simulink model "CM340A_AdcDiagc"
settings: Solver=FixedStepDiscrete  SolverMode=SingleTasking  StartTime=0.0  StopTime=1  FixedStep=0.002  RelTol=1e-3
values from neighbouring files (symbols this model uses):
  Adc0Diagc = DataDict.NTC    [CM340A_AdcDiagc_DataDict.m]
  Adc1Diagc = DataDict.NTC    [CM340A_AdcDiagc_DataDict.m]
  ADCDIAG0REFVOLT_VOLT_F32 = DataDict.Constant    [CM340A_AdcDiagc_DataDict.m]
  ADCDIAG2REFVOLT_VOLT_F32 = DataDict.Constant    [CM340A_AdcDiagc_DataDict.m]
  ADCDIAG4REFVOLT_VOLT_F32 = DataDict.Constant    [CM340A_AdcDiagc_DataDict.m]
  AdcDiagcNtc0x032FailStep = DataDict.Calibration    [CM340A_AdcDiagc_DataDict.m]
  AdcDiagcNtc0x032PassStep = DataDict.Calibration    [CM340A_AdcDiagc_DataDict.m]
  AdcDiagcNtc0x033FailStep = DataDict.Calibration    [CM340A_AdcDiagc_DataDict.m]
  AdcDiagcNtc0x033PassStep = DataDict.Calibration    [CM340A_AdcDiagc_DataDict.m]
  AdcDiagcSt = DataDict.PIM    [CM340A_AdcDiagc_DataDict.m]
  ADCDIAGPARFLTPRM_CNT_U08 = DataDict.Constant    [CM340A_AdcDiagc_DataDict.m]
  ADCDIAGSCANGROUP2REFFLTPRM_CNT_U08 = DataDict.Constant    [CM340A_AdcDiagc_DataDict.m]
  ADCDIAGSCANGROUP3REFFLTPRM_CNT_U08 = DataDict.Constant    [CM340A_AdcDiagc_DataDict.m]
  ADCDIAGSCANGROUPENDREFVOLT_VOLT_F32 = DataDict.Constant    [CM340A_AdcDiagc_DataDict.m]
  ADCDIAGSCANGROUPSTRTREFVOLT_VOLT_F32 = DataDict.Constant    [CM340A_AdcDiagc_DataDict.m]
  ADCDNECRPARERRCLR_CNT_U08 = DataDict.Constant    [CM340A_AdcDiagc_DataDict.m]
  ADCDNPERPARERRMASK_CNT_U08 = DataDict.Constant    [CM340A_AdcDiagc_DataDict.m]
  VIRTCH21_CNT_U08 = DataDict.Constant    [CM340A_AdcDiagc_DataDict.m]
  VIRTCH22_CNT_U08 = DataDict.Constant    [CM340A_AdcDiagc_DataDict.m]
  VIRTCH23_CNT_U08 = DataDict.Constant    [CM340A_AdcDiagc_DataDict.m]
undefined symbols (not defined in the file or in its folder): NtcSts1, sigbuilder_block, SigQlfr1
libraries: simulink x42, CM340A_AdcDiagc_Library x40
(part 2 of 4)

== system CM340A_AdcDiagc/AdcDiagc/AdcDiagcPer1/NTC Fault Processing1 ==
  Adc1ParFlt : Inport
  Adc1 ParmByte : Inport  Port=2
  Add : Sum
  Atomic Subsystem : Subsystem  RequirementInfo="{'linktype_rmi_doors' '000079f2 (/ESG Group/FDD Module Requirements/EA4 Specific/CM340A_AdcDiagc)' '#CM340A_134' 'true' 'REQ:  CM340A_134' '' ; 'linktype_rmi_doors' '000079f2 (/ESG Group/FDD Module Requirements/EA4 Specific/CM340A_AdcDiagc)' '#CM340A_136' 'true' 'REQ:  CM340A_136' '' } %GIDa_bde32a42_2438_4464_b67f_8e12736c6683"  TreatAsAtomicUnit=on
  Constant3 : Constant  Value=Adc1Diagc
  CopyRight2 : Subsystem  Description=|  mask(Copyright Information){none=on}
      | Copyright info block.                                               
      |                                                                     
      | Place copyright information at the top of every subsystem in design.
      mask prompts: none "No parameters"
      mask help: Place copyright information at the top of every subsystem in design.
      mask Display:
      | NxtrConf = 'Nexteer Confidential';
      | 
      | sys = bdroot; %handle for the current model ("system")
      | first = get_param(sys,'Created');
      | first = first(end-3:end);  %year is last four digits
      | 
      | last = get_param(sys,'LastModifiedDate');
      | if isempty(last)
      |     last = datestr(now,'yyyy');
      | else
      |     last = last(end-3:end);
      | end
      | 
      | if strcmp(first,last)
      |     fprintf('%s -- Copyright %s Nexteer',NxtrConf,first)
      | else
      |     fprintf('%s -- %s%s- %s Nexteer',NxtrConf,char(169),first,last)
      | end
  Data Type Conversion : DataTypeConversion  OutDataTypeStr=Enum: SigQlfr1
  Data Type Conversion1 : DataTypeConversion  OutDataTypeStr=uint8
  Enumerated Constant : simulink/Sources/Enumerated Constant  OutDataTypeStr=Enum: SigQlfr1  Value=SigQlfr1.SIGQLFR_FAILD  SampleTime=inf
  GetNtcQlfr : Subsystem  RequirementInfo={} %GIDa_4498a704_80e4_4371_b34d_a62039516cac
  Relational Operator : RelationalOperator  Operator===  OutDataTypeStr=boolean
  SetNtcSts : Subsystem  RequirementInfo="{'linktype_rmi_doors' '000079f2 (/ESG Group/FDD Module Requirements/EA4 Specific/CM340A_AdcDiagc)' '#CM340A_130' 'true' 'REQ:  CM340A_130' '' } %GIDa_b72dd821_a9e1_4e8a_8139_63a1f2cdcabd"
  Adc1Faild : Outport
  wires:
  Relational Operator/1 -> Adc1Faild/1
  Enumerated Constant/1 -> Relational Operator/2
  Data Type Conversion/1 -> Relational Operator/1
  GetNtcQlfr/1(NtcQlfr) -> Data Type Conversion1/1
  Adc1 ParmByte/1 -> Add/1
  Atomic Subsystem/2(DebStep) -> SetNtcSts/4(DebStep)
  Atomic Subsystem/1(NtcSts) -> SetNtcSts/3(NtcSts)
  Constant3/1 -> GetNtcQlfr/1(NtcNr), SetNtcSts/1(NtcNr)  "NtcNr"
  Data Type Conversion1/1 -> Data Type Conversion/1
  Adc1ParFlt/1 -> Add/2
  Add/1 -> SetNtcSts/2(NtcStInfo), Atomic Subsystem/1(NtcStInfo)

== system CM340A_AdcDiagc/AdcDiagc/AdcDiagcPer1/Adc Daigc Pointer/CopyRight2 ==

== system CM340A_AdcDiagc/AdcDiagc/AdcDiagcPer1/Adc Daigc Pointer/Strt & End Ptr Output ==
  CopyRight2 : Subsystem  Description=|  mask(Copyright Information){none=on}
      | Copyright info block.                                               
      |                                                                     
      | Place copyright information at the top of every subsystem in design.
      mask prompts: none "No parameters"
      mask help: Place copyright information at the top of every subsystem in design.
      mask Display:
      | NxtrConf = 'Nexteer Confidential';
      | 
      | sys = bdroot; %handle for the current model ("system")
      | first = get_param(sys,'Created');
      | first = first(end-3:end);  %year is last four digits
      | 
      | last = get_param(sys,'LastModifiedDate');
      | if isempty(last)
      |     last = datestr(now,'yyyy');
      | else
      |     last = last(end-3:end);
      | end
      | 
      | if strcmp(first,last)
      |     fprintf('%s -- Copyright %s Nexteer',NxtrConf,first)
      | else
      |     fprintf('%s -- %s%s- %s Nexteer',NxtrConf,char(169),first,last)
      | end
  Data Store Read : DataStoreRead  DataStoreName=AdcDiagcStrtPtr
  Data Store Read1 : DataStoreRead  DataStoreName=AdcDiagcEndPtr
  AdcDiagcStrtPtr : Outport
  AdcDiagcEndPtr : Outport  Port=2
  wires:
  Data Store Read/1 -> AdcDiagcStrtPtr/1
  Data Store Read1/1 -> AdcDiagcEndPtr/1

== system CM340A_AdcDiagc/AdcDiagc/AdcDiagcPer1/Adc Daigc Pointer/Strt & End Ptr Store ==
  Adc Diag State : Inport
  CopyRight2 : Subsystem  Description=|  mask(Copyright Information){none=on}
      | Copyright info block.                                               
      |                                                                     
      | Place copyright information at the top of every subsystem in design.
      mask prompts: none "No parameters"
      mask help: Place copyright information at the top of every subsystem in design.
      mask Display:
      | NxtrConf = 'Nexteer Confidential';
      | 
      | sys = bdroot; %handle for the current model ("system")
      | first = get_param(sys,'Created');
      | first = first(end-3:end);  %year is last four digits
      | 
      | last = get_param(sys,'LastModifiedDate');
      | if isempty(last)
      |     last = datestr(now,'yyyy');
      | else
      |     last = last(end-3:end);
      | end
      | 
      | if strcmp(first,last)
      |     fprintf('%s -- Copyright %s Nexteer',NxtrConf,first)
      | else
      |     fprintf('%s -- %s%s- %s Nexteer',NxtrConf,char(169),first,last)
      | end
  Data Store Write : DataStoreWrite  DataStoreName=AdcDiagcStrtPtr
  Data Store Write1 : DataStoreWrite  DataStoreName=AdcDiagcEndPtr
  Merge : Merge  Inputs=4
  Merge1 : Merge  Inputs=4
  State 0 : Subsystem  RequirementInfo="{'linktype_rmi_doors' '000079f2 (/ESG Group/FDD Module Requirements/EA4 Specific/CM340A_AdcDiagc)' '#CM340A_189' 'true' 'REQ:  CM340A_189' '' } %GIDa_d7231089_39f2_44f7_8ddf_68c1ec68f84f"  TreatAsAtomicUnit=on
  State 1 : Subsystem  RequirementInfo="{'linktype_rmi_doors' '000079f2 (/ESG Group/FDD Module Requirements/EA4 Specific/CM340A_AdcDiagc)' '#CM340A_115' 'true' 'REQ:  CM340A_115' '' } %GIDa_53ce9ffd_18d8_43bb_bb31_5668534b0a0e"  TreatAsAtomicUnit=on
  State 2 : Subsystem  RequirementInfo="{'linktype_rmi_doors' '000079f2 (/ESG Group/FDD Module Requirements/EA4 Specific/CM340A_AdcDiagc)' '#CM340A_96' 'true' 'REQ:  CM340A_96' '' } %GIDa_d0356ceb_c141_4346_a11e_a54c0b3cccc5"  TreatAsAtomicUnit=on
  State 4 : Subsystem  RequirementInfo="{'linktype_rmi_doors' '000079f2 (/ESG Group/FDD Module Requirements/EA4 Specific/CM340A_AdcDiagc)' '#CM340A_106' 'true' 'REQ:  CM340A_106' '' } %GIDa_e4830bd7_ebc0_413b_b5ae_d9af4b1dd5b0"  TreatAsAtomicUnit=on
  State 6 : Subsystem  RequirementInfo="{'linktype_rmi_doors' '000079f2 (/ESG Group/FDD Module Requirements/EA4 Specific/CM340A_AdcDiagc)' '#CM340A_115' 'true' 'REQ:  CM340A_115' '' } %GIDa_697a9f40_2b37_43b7_b3e2_4ac1a7799fac"  TreatAsAtomicUnit=on
  State Based Determination1 : If  IfExpression=u1 == 0  ElseIfExpressions=u1 == 2, u1 == 4, u1 == 6
  wires:
  State Based Determination1/4 -> State 6/Action
  State 4/1(AdcDiagcStrtPtr) -> Merge/3
  State Based Determination1/1 -> State 0/Action
  State 0/1(AdcDiagcStrtPtr) -> Merge/1
  State Based Determination1/2 -> State 2/Action
  State 6/1(AdcDiagcStrtPtr) -> Merge/4
  Adc Diag State/1 -> State Based Determination1/1
  State 6/2(AdcDiagcEndPtr) -> Merge1/4
  Merge1/1 -> Data Store Write1/1
  State 2/1(AdcDiagcStrtPtr) -> Merge/2
  State 0/2(AdcDiagcEndPtr) -> Merge1/1
  State Based Determination1/3 -> State 4/Action
  Merge/1 -> Data Store Write/1
  State 2/2(AdcDiagcEndPtr) -> Merge1/2
  State 4/2(AdcDiagcEndPtr) -> Merge1/3
  State Based Determination1/5 -> State 1/Action

== system CM340A_AdcDiagc/AdcDiagc/AdcDiagcPer1/Adc Diag State/CopyRight2 ==

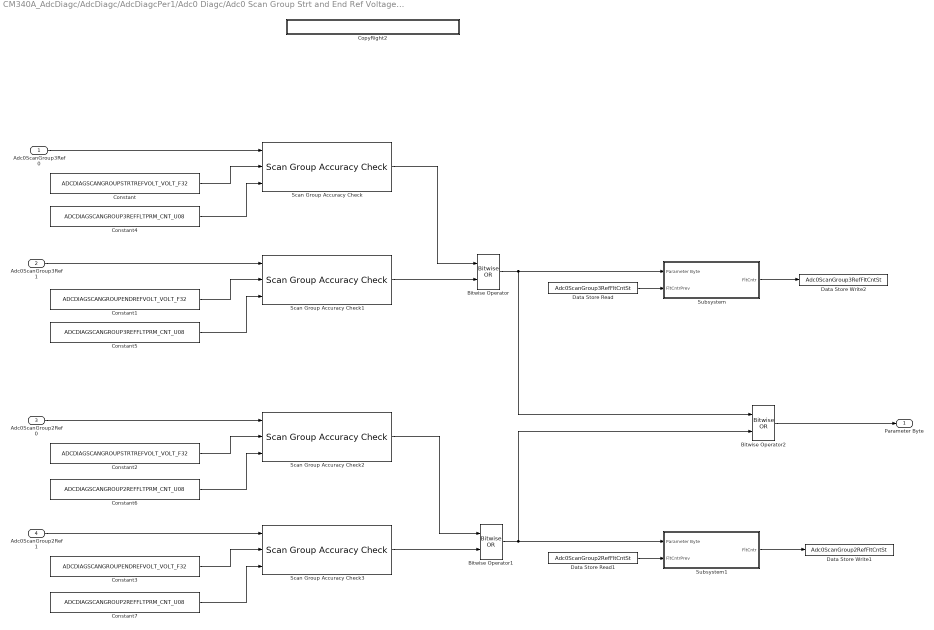
== system CM340A_AdcDiagc/AdcDiagc/AdcDiagcPer1/Adc0 Diagc/Adc0 Scan Group Strt and End Ref Voltage Diagc ==
  Adc0ScanGroup3Ref0 : Inport  RequirementInfo={} %GIDa_3923f31e_b6aa_43ec_bc9b_c94f6f317497
  Adc0ScanGroup3Ref1 : Inport  RequirementInfo={} %GIDa_ba8bf00c_f3fc_40d7_abef_0dabf128981a  Port=2
  Adc0ScanGroup2Ref0 : Inport  RequirementInfo={} %GIDa_6ca5502f_1ae3_4ae8_b00c_fe0941fa35eb  Port=3
  Adc0ScanGroup2Ref1 : Inport  RequirementInfo={} %GIDa_ae2e7cb2_cc28_4345_abb7_491be77205bd  Port=4
  Bitwise Operator : simulink/Logic and Bit Operations/Bitwise Operator  logicop=OR  UseBitMask=off  NumInputPorts=2  BitMask=bin2dec('11011001')  BitMaskRealWorld=Stored Integer
  Bitwise Operator1 : simulink/Logic and Bit Operations/Bitwise Operator  logicop=OR  UseBitMask=off  NumInputPorts=2  BitMask=bin2dec('11011001')  BitMaskRealWorld=Stored Integer
  Bitwise Operator2 : simulink/Logic and Bit Operations/Bitwise Operator  logicop=OR  UseBitMask=off  NumInputPorts=2  BitMask=bin2dec('11011001')  BitMaskRealWorld=Stored Integer
  Constant : Constant  Value=ADCDIAGSCANGROUPSTRTREFVOLT_VOLT_F32
  Constant1 : Constant  Value=ADCDIAGSCANGROUPENDREFVOLT_VOLT_F32
  Constant2 : Constant  Value=ADCDIAGSCANGROUPSTRTREFVOLT_VOLT_F32
  Constant3 : Constant  Value=ADCDIAGSCANGROUPENDREFVOLT_VOLT_F32
  Constant4 : Constant  Value=ADCDIAGSCANGROUP3REFFLTPRM_CNT_U08  OutDataTypeStr=uint8
  Constant5 : Constant  Value=ADCDIAGSCANGROUP3REFFLTPRM_CNT_U08  OutDataTypeStr=uint8
  Constant6 : Constant  Value=ADCDIAGSCANGROUP2REFFLTPRM_CNT_U08  OutDataTypeStr=uint8
  Constant7 : Constant  Value=ADCDIAGSCANGROUP2REFFLTPRM_CNT_U08  OutDataTypeStr=uint8
  CopyRight2 : Subsystem  Description=|  mask(Copyright Information){none=on}
      | Copyright info block.                                               
      |                                                                     
      | Place copyright information at the top of every subsystem in design.
      mask prompts: none "No parameters"
      mask help: Place copyright information at the top of every subsystem in design.
      mask Display:
      | NxtrConf = 'Nexteer Confidential';
      | 
      | sys = bdroot; %handle for the current model ("system")
      | first = get_param(sys,'Created');
      | first = first(end-3:end);  %year is last four digits
      | 
      | last = get_param(sys,'LastModifiedDate');
      | if isempty(last)
      |     last = datestr(now,'yyyy');
      | else
      |     last = last(end-3:end);
      | end
      | 
      | if strcmp(first,last)
      |     fprintf('%s -- Copyright %s Nexteer',NxtrConf,first)
      | else
      |     fprintf('%s -- %s%s- %s Nexteer',NxtrConf,char(169),first,last)
      | end
  Data Store Read : DataStoreRead  DataStoreName=Adc0ScanGroup3RefFltCntSt
  Data Store Read1 : DataStoreRead  DataStoreName=Adc0ScanGroup2RefFltCntSt
  Data Store Write1 : DataStoreWrite  DataStoreName=Adc0ScanGroup2RefFltCntSt
  Data Store Write2 : DataStoreWrite  DataStoreName=Adc0ScanGroup3RefFltCntSt
  Scan Group Accuracy Check{,1..3} (4 alike) : CM340A_AdcDiagc_Library/Scan Group Accuracy Check
  Subsystem : Subsystem
  Subsystem1 : Subsystem
  Parameter Byte : Outport
  wires:
  Adc0ScanGroup3Ref0/1 -> Scan Group Accuracy Check/1
  Constant/1 -> Scan Group Accuracy Check/2
  Adc0ScanGroup3Ref1/1 -> Scan Group Accuracy Check1/1
  Constant1/1 -> Scan Group Accuracy Check1/2
  Adc0ScanGroup2Ref0/1 -> Scan Group Accuracy Check2/1
  Constant2/1 -> Scan Group Accuracy Check2/2
  Scan Group Accuracy Check/1 -> Bitwise Operator/1
  Scan Group Accuracy Check1/1 -> Bitwise Operator/2
  Bitwise Operator/1 -> Bitwise Operator2/1, Subsystem/1(Parameter Byte)
  Adc0ScanGroup2Ref1/1 -> Scan Group Accuracy Check3/1
  Constant3/1 -> Scan Group Accuracy Check3/2
  Scan Group Accuracy Check3/1 -> Bitwise Operator1/2
  Bitwise Operator2/1 -> Parameter Byte/1
  Scan Group Accuracy Check2/1 -> Bitwise Operator1/1
  Constant4/1 -> Scan Group Accuracy Check/3
  Constant5/1 -> Scan Group Accuracy Check1/3
  Constant6/1 -> Scan Group Accuracy Check2/3
  Constant7/1 -> Scan Group Accuracy Check3/3
  Subsystem/1(FltCntr) -> Data Store Write2/1
  Bitwise Operator1/1 -> Subsystem1/1(Parameter Byte), Bitwise Operator2/2
  Data Store Read/1 -> Subsystem/2(FltCntrPrev)
  Data Store Read1/1 -> Subsystem1/2(FltCntrPrev)
  Subsystem1/1(FltCntr) -> Data Store Write1/1

== system CM340A_AdcDiagc/AdcDiagc/AdcDiagcPer1/Adc0 Diagc/CopyRight2 ==

== system CM340A_AdcDiagc/AdcDiagc/AdcDiagcPer1/Adc0 Diagc/State 0, 2, 4, 6 ==
  Adc0SelfDiag0 : Inport  RequirementInfo={} %GIDa_94e29999_33ff_4201_8add_daa4f5d70819
  Adc0SelfDiag2 : Inport  RequirementInfo={} %GIDa_c26eddb7_e945_49bf_b8c5_dde3d8ca2d62  Port=2
  Adc0SelfDiag4 : Inport  RequirementInfo={} %GIDa_06c9974f_8877_4a3b_918f_cfd71e4c9c58  Port=3
  Adc0DiagSt : Inport  RequirementInfo={} %GIDa_3045ed8c_f79b_488d_b603_a76a50a7acd0  Port=4
  Action Port : ActionPort  ActionType=case
  Merge : Merge  Inputs=4
  State 0 : Subsystem  RequirementInfo="{'linktype_rmi_doors' '000079f2 (/ESG Group/FDD Module Requirements/EA4 Specific/CM340A_AdcDiagc)' '#CM340A_189' 'true' 'REQ:  CM340A_189' '' } %GIDa_a6da38dc_83ca_4031_acbe_834917661ebd"  TreatAsAtomicUnit=on
  State 2 : Subsystem  RequirementInfo="{'linktype_rmi_doors' '000079f2 (/ESG Group/FDD Module Requirements/EA4 Specific/CM340A_AdcDiagc)' '#CM340A_96' 'true' 'REQ:  CM340A_96' '' } %GIDa_33825e2f_213e_4946_b631_0cc3f71b8274"  TreatAsAtomicUnit=on
  State 4 : Subsystem  RequirementInfo="{'linktype_rmi_doors' '000079f2 (/ESG Group/FDD Module Requirements/EA4 Specific/CM340A_AdcDiagc)' '#CM340A_106' 'true' 'REQ:  CM340A_106' '' } %GIDa_cf9e8958_cd24_4cdd_ad67_cff793a850a5"  TreatAsAtomicUnit=on
  State 6 : Subsystem  RequirementInfo="{'linktype_rmi_doors' '000079f2 (/ESG Group/FDD Module Requirements/EA4 Specific/CM340A_AdcDiagc)' '#CM340A_115' 'true' 'REQ:  CM340A_115' '' } %GIDa_c79baab0_0759_49b6_a0c6_0635325daffc"  TreatAsAtomicUnit=on
  State Based Determination : If  IfExpression=u1 == 0  ElseIfExpressions=u1 == 2, u1 == 4
  Parameter Byte : Outport
  wires:
  Adc0DiagSt/1 -> State 2/4(DiagState), State 6/4(DiagState), State 4/4(DiagState), State 0/4(DiagState), State Based Determination/1
  Adc0SelfDiag0/1 -> State 6/1(Adc0SelfDiag0), State 4/1(Adc0SelfDiag0), State 2/1(Adc0SelfDiag0), State 0/1(Adc0SelfDiag0)
  Adc0SelfDiag2/1 -> State 6/2(Adc0SelfDiag2), State 4/2(Adc0SelfDiag2), State 2/2(Adc0SelfDiag2), State 0/2(Adc0SelfDiag2)
  Adc0SelfDiag4/1 -> State 6/3(Adc0SelfDiag4), State 4/3(Adc0SelfDiag4), State 2/3(Adc0SelfDiag4), State 0/3(Adc0SelfDiag4)
  State 0/1(Parameter Byte) -> Merge/1
  State 2/1(Parameter Byte) -> Merge/2
  State 4/1(Parameter Byte) -> Merge/3
  State 6/1(Parameter Byte) -> Merge/4
  Merge/1 -> Parameter Byte/1
  State Based Determination/1 -> State 0/Action
  State Based Determination/2 -> State 2/Action
  State Based Determination/3 -> State 4/Action
  State Based Determination/4 -> State 6/Action

== system CM340A_AdcDiagc/AdcDiagc/AdcDiagcPer1/Adc0 Diagc/State 1,3,5,7 ==
  Action Port : ActionPort  ActionType=default
  Constant : Constant  Value=0  OutDataTypeStr=uint8
  CopyRight2 : Subsystem  Description=|  mask(Copyright Information){none=on}
      | Copyright info block.                                               
      |                                                                     
      | Place copyright information at the top of every subsystem in design.
      mask prompts: none "No parameters"
      mask help: Place copyright information at the top of every subsystem in design.
      mask Display:
      | NxtrConf = 'Nexteer Confidential';
      | 
      | sys = bdroot; %handle for the current model ("system")
      | first = get_param(sys,'Created');
      | first = first(end-3:end);  %year is last four digits
      | 
      | last = get_param(sys,'LastModifiedDate');
      | if isempty(last)
      |     last = datestr(now,'yyyy');
      | else
      |     last = last(end-3:end);
      | end
      | 
      | if strcmp(first,last)
      |     fprintf('%s -- Copyright %s Nexteer',NxtrConf,first)
      | else
      |     fprintf('%s -- %s%s- %s Nexteer',NxtrConf,char(169),first,last)
      | end
  Parameter Byte : Outport
  wires:
  Constant/1 -> Parameter Byte/1

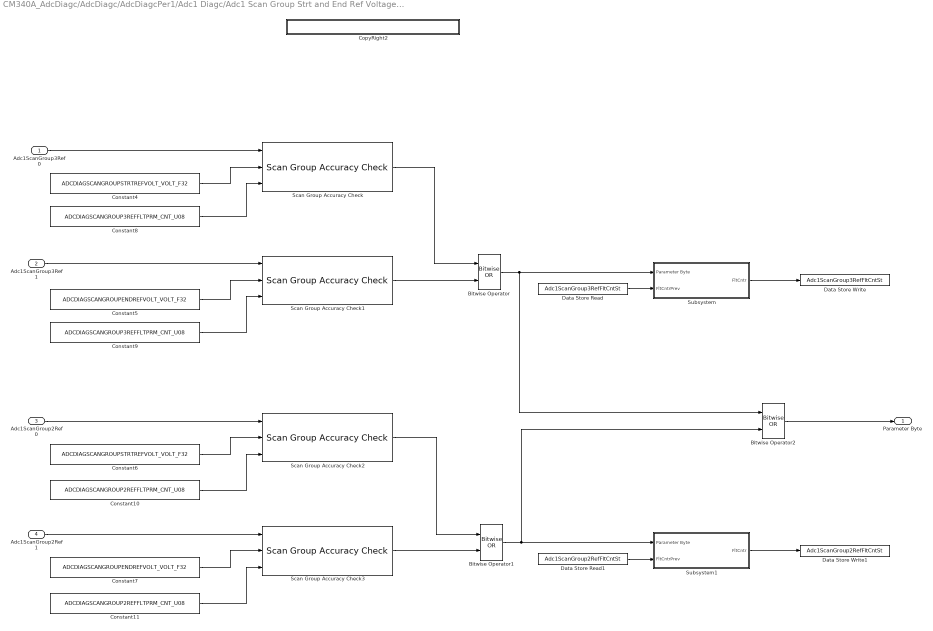
== system CM340A_AdcDiagc/AdcDiagc/AdcDiagcPer1/Adc1 Diagc/Adc1 Scan Group Strt and End Ref Voltage Diagc ==
  Adc1ScanGroup3Ref0 : Inport  RequirementInfo={} %GIDa_01845f96_04cc_48cb_8cdf_d81f529bf610
  Adc1ScanGroup3Ref1 : Inport  RequirementInfo={} %GIDa_d1be0a00_9783_4d18_831d_acb83b27fe4f  Port=2
  Adc1ScanGroup2Ref0 : Inport  RequirementInfo={} %GIDa_3fed8bb6_e00c_497f_b5bc_7887f6a81f53  Port=3
  Adc1ScanGroup2Ref1 : Inport  RequirementInfo={} %GIDa_4db4f757_00a1_4030_b70d_cb6c9e614cb5  Port=4
  Bitwise Operator : simulink/Logic and Bit Operations/Bitwise Operator  logicop=OR  UseBitMask=off  NumInputPorts=2  BitMask=bin2dec('11011001')  BitMaskRealWorld=Stored Integer
  Bitwise Operator1 : simulink/Logic and Bit Operations/Bitwise Operator  logicop=OR  UseBitMask=off  NumInputPorts=2  BitMask=bin2dec('11011001')  BitMaskRealWorld=Stored Integer
  Bitwise Operator2 : simulink/Logic and Bit Operations/Bitwise Operator  logicop=OR  UseBitMask=off  NumInputPorts=2  BitMask=bin2dec('11011001')  BitMaskRealWorld=Stored Integer
  Constant10 : Constant  Value=ADCDIAGSCANGROUP2REFFLTPRM_CNT_U08  OutDataTypeStr=uint8
  Constant11 : Constant  Value=ADCDIAGSCANGROUP2REFFLTPRM_CNT_U08  OutDataTypeStr=uint8
  Constant4 : Constant  Value=ADCDIAGSCANGROUPSTRTREFVOLT_VOLT_F32
  Constant5 : Constant  Value=ADCDIAGSCANGROUPENDREFVOLT_VOLT_F32
  Constant6 : Constant  Value=ADCDIAGSCANGROUPSTRTREFVOLT_VOLT_F32
  Constant7 : Constant  Value=ADCDIAGSCANGROUPENDREFVOLT_VOLT_F32
  Constant8 : Constant  Value=ADCDIAGSCANGROUP3REFFLTPRM_CNT_U08  OutDataTypeStr=uint8
  Constant9 : Constant  Value=ADCDIAGSCANGROUP3REFFLTPRM_CNT_U08  OutDataTypeStr=uint8
  CopyRight2 : Subsystem  Description=|  mask(Copyright Information){none=on}
      | Copyright info block.                                               
      |                                                                     
      | Place copyright information at the top of every subsystem in design.
      mask prompts: none "No parameters"
      mask help: Place copyright information at the top of every subsystem in design.
      mask Display:
      | NxtrConf = 'Nexteer Confidential';
      | 
      | sys = bdroot; %handle for the current model ("system")
      | first = get_param(sys,'Created');
      | first = first(end-3:end);  %year is last four digits
      | 
      | last = get_param(sys,'LastModifiedDate');
      | if isempty(last)
      |     last = datestr(now,'yyyy');
      | else
      |     last = last(end-3:end);
      | end
      | 
      | if strcmp(first,last)
      |     fprintf('%s -- Copyright %s Nexteer',NxtrConf,first)
      | else
      |     fprintf('%s -- %s%s- %s Nexteer',NxtrConf,char(169),first,last)
      | end
  Data Store Read : DataStoreRead  DataStoreName=Adc1ScanGroup3RefFltCntSt
  Data Store Read1 : DataStoreRead  DataStoreName=Adc1ScanGroup2RefFltCntSt
  Data Store Write : DataStoreWrite  DataStoreName=Adc1ScanGroup3RefFltCntSt
  Data Store Write1 : DataStoreWrite  DataStoreName=Adc1ScanGroup2RefFltCntSt
  Scan Group Accuracy Check{,1..3} (4 alike) : CM340A_AdcDiagc_Library/Scan Group Accuracy Check
  Subsystem : Subsystem
  Subsystem1 : Subsystem
  Parameter Byte : Outport
  wires:
  Scan Group Accuracy Check/1 -> Bitwise Operator/1
  Scan Group Accuracy Check1/1 -> Bitwise Operator/2
  Subsystem/1(FltCntr) -> Data Store Write/1
  Scan Group Accuracy Check2/1 -> Bitwise Operator1/1
  Scan Group Accuracy Check3/1 -> Bitwise Operator1/2
  Subsystem1/1(FltCntr) -> Data Store Write1/1
  Bitwise Operator2/1 -> Parameter Byte/1
  Adc1ScanGroup3Ref0/1 -> Scan Group Accuracy Check/1
  Constant4/1 -> Scan Group Accuracy Check/2
  Adc1ScanGroup3Ref1/1 -> Scan Group Accuracy Check1/1
  Constant5/1 -> Scan Group Accuracy Check1/2
  Adc1ScanGroup2Ref0/1 -> Scan Group Accuracy Check2/1
  Constant6/1 -> Scan Group Accuracy Check2/2
  Adc1ScanGroup2Ref1/1 -> Scan Group Accuracy Check3/1
  Constant7/1 -> Scan Group Accuracy Check3/2
  Constant8/1 -> Scan Group Accuracy Check/3
  Constant9/1 -> Scan Group Accuracy Check1/3
  Constant10/1 -> Scan Group Accuracy Check2/3
  Constant11/1 -> Scan Group Accuracy Check3/3
  Bitwise Operator/1 -> Subsystem/1(Parameter Byte), Bitwise Operator2/1
  Bitwise Operator1/1 -> Subsystem1/1(Parameter Byte), Bitwise Operator2/2
  Data Store Read/1 -> Subsystem/2(FltCntrPrev)
  Data Store Read1/1 -> Subsystem1/2(FltCntrPrev)

== system CM340A_AdcDiagc/AdcDiagc/AdcDiagcPer1/Adc1 Diagc/CopyRight2 ==

== system CM340A_AdcDiagc/AdcDiagc/AdcDiagcPer1/Adc1 Diagc/State 0,2,4,6 ==
  Adc1SelfDiag0 : Inport  RequirementInfo={} %GIDa_34a48fa0_dd63_46cc_bd9d_829bbe1f86cf
  Adc1SelfDiag2 : Inport  RequirementInfo={} %GIDa_4de6ae8c_be2f_440b_b497_7b7a185d7705  Port=2
  Adc1SelfDiag4 : Inport  RequirementInfo={} %GIDa_eacb0038_7c4f_43e2_bdc2_c657f83f78ba  Port=3
  Adc1DiagSt : Inport  RequirementInfo={} %GIDa_82c28b46_226d_4e6c_8857_1d9eb21c6cb5  Port=4
  Action Port : ActionPort  ActionType=case
  CopyRight2 : Subsystem  Description=|  mask(Copyright Information){none=on}
      | Copyright info block.                                               
      |                                                                     
      | Place copyright information at the top of every subsystem in design.
      mask prompts: none "No parameters"
      mask help: Place copyright information at the top of every subsystem in design.
      mask Display:
      | NxtrConf = 'Nexteer Confidential';
      | 
      | sys = bdroot; %handle for the current model ("system")
      | first = get_param(sys,'Created');
      | first = first(end-3:end);  %year is last four digits
      | 
      | last = get_param(sys,'LastModifiedDate');
      | if isempty(last)
      |     last = datestr(now,'yyyy');
      | else
      |     last = last(end-3:end);
      | end
      | 
      | if strcmp(first,last)
      |     fprintf('%s -- Copyright %s Nexteer',NxtrConf,first)
      | else
      |     fprintf('%s -- %s%s- %s Nexteer',NxtrConf,char(169),first,last)
      | end
  Merge : Merge  Inputs=4
  State 0 : Subsystem  RequirementInfo="{'linktype_rmi_doors' '000079f2 (/ESG Group/FDD Module Requirements/EA4 Specific/CM340A_AdcDiagc)' '#CM340A_200' 'true' 'REQ:  CM340A_200' '' } %GIDa_e35781c5_1e91_4292_ba5d_515a26f8b285"  TreatAsAtomicUnit=on
  State 2 : Subsystem  RequirementInfo="{'linktype_rmi_doors' '000079f2 (/ESG Group/FDD Module Requirements/EA4 Specific/CM340A_AdcDiagc)' '#CM340A_151' 'true' 'REQ:  CM340A_151' '' } %GIDa_47bc9f9e_be13_46f9_a398_ba75de96ec4b"  TreatAsAtomicUnit=on
  State 4 : Subsystem  RequirementInfo="{'linktype_rmi_doors' '000079f2 (/ESG Group/FDD Module Requirements/EA4 Specific/CM340A_AdcDiagc)' '#CM340A_160' 'true' 'REQ:  CM340A_160' '' } %GIDa_c894ce70_8a7d_498e_8eac_cd0715dd161e"  TreatAsAtomicUnit=on
  State 6 : Subsystem  RequirementInfo="{'linktype_rmi_doors' '000079f2 (/ESG Group/FDD Module Requirements/EA4 Specific/CM340A_AdcDiagc)' '#CM340A_169' 'true' 'REQ:  CM340A_169' '' } %GIDa_9580dbab_c802_4d44_ba6f_46aa79aa5561"  TreatAsAtomicUnit=on
  State Based Determination : If  IfExpression=u1 == 0  ElseIfExpressions=u1 == 2, u1 == 4
  Parameter Byte : Outport
  wires:
  Merge/1 -> Parameter Byte/1
  State 6/1(Parameter Byte) -> Merge/4
  State 4/1(Parameter Byte) -> Merge/3
  State 2/1(Parameter Byte) -> Merge/2
  State 0/1(Parameter Byte) -> Merge/1
  Adc1SelfDiag4/1 -> State 6/3(Adc1SelfDiag4), State 4/3(Adc1SelfDiag4), State 2/3(Adc1SelfDiag4), State 0/3(Adc1SelfDiag4)
  Adc1SelfDiag2/1 -> State 6/2(Adc1SelfDiag2), State 4/2(Adc1SelfDiag2), State 2/2(Adc1SelfDiag2), State 0/2(Adc1SelfDiag2)
  Adc1SelfDiag0/1 -> State 6/1(Adc1SelfDiag0), State 4/1(Adc1SelfDiag0), State 2/1(Adc1SelfDiag0), State 0/1(Adc1SelfDiag0)
  Adc1DiagSt/1 -> State 4/4(DiagState), State 6/4(DiagState), State 2/4(DiagState), State 0/4(DiagState), State Based Determination/1
  State Based Determination/1 -> State 0/Action
  State Based Determination/2 -> State 2/Action
  State Based Determination/3 -> State 4/Action
  State Based Determination/4 -> State 6/Action

== system CM340A_AdcDiagc/AdcDiagc/AdcDiagcPer1/Adc1 Diagc/State 1,3,5,7 ==
  Action Port : ActionPort  ActionType=default
  Constant : Constant  Value=0  OutDataTypeStr=uint8
  CopyRight2 : Subsystem  Description=|  mask(Copyright Information){none=on}
      | Copyright info block.                                               
      |                                                                     
      | Place copyright information at the top of every subsystem in design.
      mask prompts: none "No parameters"
      mask help: Place copyright information at the top of every subsystem in design.
      mask Display:
      | NxtrConf = 'Nexteer Confidential';
      | 
      | sys = bdroot; %handle for the current model ("system")
      | first = get_param(sys,'Created');
      | first = first(end-3:end);  %year is last four digits
      | 
      | last = get_param(sys,'LastModifiedDate');
      | if isempty(last)
      |     last = datestr(now,'yyyy');
      | else
      |     last = last(end-3:end);
      | end
      | 
      | if strcmp(first,last)
      |     fprintf('%s -- Copyright %s Nexteer',NxtrConf,first)
      | else
      |     fprintf('%s -- %s%s- %s Nexteer',NxtrConf,char(169),first,last)
      | end
  Parameter Byte : Outport
  wires:
  Constant/1 -> Parameter Byte/1

== system CM340A_AdcDiagc/AdcDiagc/AdcDiagcPer1/AdcDiagcPer2/CopyRight2 ==

== system CM340A_AdcDiagc/AdcDiagc/AdcDiagcPer1/AdcDiagcPer2/Set Adc0ParFlt 0 ==
  Action Port : ActionPort  ActionType=else
  CopyRight2 : Subsystem  Description=|  mask(Copyright Information){none=on}
      | Copyright info block.                                               
      |                                                                     
      | Place copyright information at the top of every subsystem in design.
      mask prompts: none "No parameters"
      mask help: Place copyright information at the top of every subsystem in design.
      mask Display:
      | NxtrConf = 'Nexteer Confidential';
      | 
      | sys = bdroot; %handle for the current model ("system")
      | first = get_param(sys,'Created');
      | first = first(end-3:end);  %year is last four digits
      | 
      | last = get_param(sys,'LastModifiedDate');
      | if isempty(last)
      |     last = datestr(now,'yyyy');
      | else
      |     last = last(end-3:end);
      | end
      | 
      | if strcmp(first,last)
      |     fprintf('%s -- Copyright %s Nexteer',NxtrConf,first)
      | else
      |     fprintf('%s -- %s%s- %s Nexteer',NxtrConf,char(169),first,last)
      | end
  zero : Constant  Value=0  OutDataTypeStr=uint8
  Adc1ParFlt : Outport
  wires:
  zero/1 -> Adc1ParFlt/1

== system CM340A_AdcDiagc/AdcDiagc/AdcDiagcPer1/AdcDiagcPer2/Set Adc0ParFlt to 0 ==
  Action Port : ActionPort  ActionType=else
  CopyRight2 : Subsystem  Description=|  mask(Copyright Information){none=on}
      | Copyright info block.                                               
      |                                                                     
      | Place copyright information at the top of every subsystem in design.
      mask prompts: none "No parameters"
      mask help: Place copyright information at the top of every subsystem in design.
      mask Display:
      | NxtrConf = 'Nexteer Confidential';
      | 
      | sys = bdroot; %handle for the current model ("system")
      | first = get_param(sys,'Created');
      | first = first(end-3:end);  %year is last four digits
      | 
      | last = get_param(sys,'LastModifiedDate');
      | if isempty(last)
      |     last = datestr(now,'yyyy');
      | else
      |     last = last(end-3:end);
      | end
      | 
      | if strcmp(first,last)
      |     fprintf('%s -- Copyright %s Nexteer',NxtrConf,first)
      | else
      |     fprintf('%s -- %s%s- %s Nexteer',NxtrConf,char(169),first,last)
      | end
  zero : Constant  Value=0  OutDataTypeStr=uint8
  Adc0ParFlt : Outport
  wires:
  zero/1 -> Adc0ParFlt/1

== system CM340A_AdcDiagc/AdcDiagc/AdcDiagcPer1/AdcDiagcPer2/Set Adc0ParFlt to 128 and Err Clr Reg to 2 ==
  note: This represents a Register Write not a software Output Variable
  Action Port : ActionPort  ActionType=then
  ADCDIAGPARFLTPRM_CNT_U08 : Constant  Value=ADCDIAGPARFLTPRM_CNT_U08  OutDataTypeStr=uint8
  ADCDIAGPARFLTPRM_CNT_U1 : Constant  Value=ADCDNECRPARERRCLR_CNT_U08  OutDataTypeStr=uint8
      settings: AttributesFormatString=%<OutDataTypeStr>
  CopyRight2 : Subsystem  Description=|  mask(Copyright Information){none=on}
      | Copyright info block.                                               
      |                                                                     
      | Place copyright information at the top of every subsystem in design.
      mask prompts: none "No parameters"
      mask help: Place copyright information at the top of every subsystem in design.
      mask Display:
      | NxtrConf = 'Nexteer Confidential';
      | 
      | sys = bdroot; %handle for the current model ("system")
      | first = get_param(sys,'Created');
      | first = first(end-3:end);  %year is last four digits
      | 
      | last = get_param(sys,'LastModifiedDate');
      | if isempty(last)
      |     last = datestr(now,'yyyy');
      | else
      |     last = last(end-3:end);
      | end
      | 
      | if strcmp(first,last)
      |     fprintf('%s -- Copyright %s Nexteer',NxtrConf,first)
      | else
      |     fprintf('%s -- %s%s- %s Nexteer',NxtrConf,char(169),first,last)
      | end
  RegOutpADCD0ECR : Terminator
  Adc0ParFlt : Outport
  wires:
  ADCDIAGPARFLTPRM_CNT_U08/1 -> Adc0ParFlt/1
  ADCDIAGPARFLTPRM_CNT_U1/1 -> RegOutpADCD0ECR/1

== system CM340A_AdcDiagc/AdcDiagc/AdcDiagcPer1/AdcDiagcPer2/Set Adc1ParFlt to 128 and Err Clr Reg to 4 ==
  note: This represents a Register Write not a software Output Variable
  Action Port : ActionPort  ActionType=then
  ADCDIAGPARFLTPRM_CNT_U08 : Constant  Value=ADCDIAGPARFLTPRM_CNT_U08  OutDataTypeStr=uint8
  ADCDIAGPARFLTPRM_CNT_U1 : Constant  Value=ADCDNECRPARERRCLR_CNT_U08  OutDataTypeStr=uint8
      settings: AttributesFormatString=%<OutDataTypeStr>
  CopyRight2 : Subsystem  Description=|  mask(Copyright Information){none=on}
      | Copyright info block.                                               
      |                                                                     
      | Place copyright information at the top of every subsystem in design.
      mask prompts: none "No parameters"
      mask help: Place copyright information at the top of every subsystem in design.
      mask Display:
      | NxtrConf = 'Nexteer Confidential';
      | 
      | sys = bdroot; %handle for the current model ("system")
      | first = get_param(sys,'Created');
      | first = first(end-3:end);  %year is last four digits
      | 
      | last = get_param(sys,'LastModifiedDate');
      | if isempty(last)
      |     last = datestr(now,'yyyy');
      | else
      |     last = last(end-3:end);
      | end
      | 
      | if strcmp(first,last)
      |     fprintf('%s -- Copyright %s Nexteer',NxtrConf,first)
      | else
      |     fprintf('%s -- %s%s- %s Nexteer',NxtrConf,char(169),first,last)
      | end
  RegOutpADCD1ECR : Terminator
  Adc1ParFlt : Outport
  wires:
  ADCDIAGPARFLTPRM_CNT_U08/1 -> Adc1ParFlt/1
  ADCDIAGPARFLTPRM_CNT_U1/1 -> RegOutpADCD1ECR/1

== system CM340A_AdcDiagc/AdcDiagc/AdcDiagcPer1/NTC Fault Processing0/Atomic Subsystem ==
  NtcStInfo : Inport  OutDataTypeStr=uint8
  CopyRight2 : Subsystem  Description=|  mask(Copyright Information){none=on}
      | Copyright info block.                                               
      |                                                                     
      | Place copyright information at the top of every subsystem in design.
      mask prompts: none "No parameters"
      mask help: Place copyright information at the top of every subsystem in design.
      mask Display:
      | NxtrConf = 'Nexteer Confidential';
      | 
      | sys = bdroot; %handle for the current model ("system")
      | first = get_param(sys,'Created');
      | first = first(end-3:end);  %year is last four digits
      | 
      | last = get_param(sys,'LastModifiedDate');
      | if isempty(last)
      |     last = datestr(now,'yyyy');
      | else
      |     last = last(end-3:end);
      | end
      | 
      | if strcmp(first,last)
      |     fprintf('%s -- Copyright %s Nexteer',NxtrConf,first)
      | else
      |     fprintf('%s -- %s%s- %s Nexteer',NxtrConf,char(169),first,last)
      | end
  Fail Step : Subsystem  TreatAsAtomicUnit=on
  If : If
  Merge : Merge
  Merge1 : Merge
  Pass Step : Subsystem  RequirementInfo={} %GIDa_f2406e4f_5e57_490d_8d1c_469ab90954f0  TreatAsAtomicUnit=on
  NtcSts : Outport
  DebStep : Outport  Port=2  OutDataTypeStr=uint16
  wires:
  NtcStInfo/1 -> If/1
  If/1 -> Fail Step/Action
  If/2 -> Pass Step/Action
  Merge/1 -> DebStep/1
  Fail Step/1(NtcSts) -> Merge1/1
  Pass Step/1(NtcSts) -> Merge1/2
  Merge1/1 -> NtcSts/1
  Fail Step/2(DebStep) -> Merge/1
  Pass Step/2(DebStep) -> Merge/2

== system CM340A_AdcDiagc/AdcDiagc/AdcDiagcPer1/NTC Fault Processing0/CopyRight2 ==

== system CM340A_AdcDiagc/AdcDiagc/AdcDiagcPer1/NTC Fault Processing0/GetNtcQlfr ==
  NtcNr : Inport
  CopyRight2 : Subsystem  Description=|  mask(Copyright Information){none=on}
      | Copyright info block.                                               
      |                                                                     
      | Place copyright information at the top of every subsystem in design.
      mask prompts: none "No parameters"
      mask help: Place copyright information at the top of every subsystem in design.
      mask Display:
      | NxtrConf = 'Nexteer Confidential';
      | 
      | sys = bdroot; %handle for the current model ("system")
      | first = get_param(sys,'Created');
      | first = first(end-3:end);  %year is last four digits
      | 
      | last = get_param(sys,'LastModifiedDate');
      | if isempty(last)
      |     last = datestr(now,'yyyy');
      | else
      |     last = last(end-3:end);
      | end
      | 
      | if strcmp(first,last)
      |     fprintf('%s -- Copyright %s Nexteer',NxtrConf,first)
      | else
      |     fprintf('%s -- %s%s- %s Nexteer',NxtrConf,char(169),first,last)
      | end
  Data Store Read : DataStoreRead  DataStoreName=Adc0DynDiagcQlfr
  Terminator : Terminator
  NtcQlfr : Outport
  wires:
  NtcNr/1 -> Terminator/1
  Data Store Read/1 -> NtcQlfr/1

== system CM340A_AdcDiagc/AdcDiagc/AdcDiagcPer1/NTC Fault Processing0/SetNtcSts ==
  note: Note:
      |
      | - "ISO Fault Debounce Design" Simulink block intent to use here for Simulation purpose only. Do not Code this block
  NtcNr : Inport
  NtcStInfo : Inport  Port=2
  NtcSts : Inport  Port=3  OutDataTypeStr=Enum: NtcSts1
  DebStep : Inport  Port=4
  CopyRight2 : Subsystem  Description=|  mask(Copyright Information){none=on}
      | Copyright info block.                                               
      |                                                                     
      | Place copyright information at the top of every subsystem in design.
      mask prompts: none "No parameters"
      mask help: Place copyright information at the top of every subsystem in design.
      mask Display:
      | NxtrConf = 'Nexteer Confidential';
      | 
      | sys = bdroot; %handle for the current model ("system")
      | first = get_param(sys,'Created');
      | first = first(end-3:end);  %year is last four digits
      | 
      | last = get_param(sys,'LastModifiedDate');
      | if isempty(last)
      |     last = datestr(now,'yyyy');
      | else
      |     last = last(end-3:end);
      | end
      | 
      | if strcmp(first,last)
      |     fprintf('%s -- Copyright %s Nexteer',NxtrConf,first)
      | else
      |     fprintf('%s -- %s%s- %s Nexteer',NxtrConf,char(169),first,last)
      | end
  Data Store Write : DataStoreWrite  DataStoreName=Adc0DynDiagcQlfr
  Data Type Conversion1 : DataTypeConversion  OutMin=0  OutMax=255  OutDataTypeStr=uint8
  Enabled Subsystem : Subsystem  TreatAsAtomicUnit=on
  Faild : Constant  Value=2
  Ground : Ground
  ISO Fault Debounce Design : Stateflow chart  TreatAsAtomicUnit=on
      settings: AttributesFormatString=|
      | Simulation Purpose Only.
      | Do Not Code this block
      | Diagnostic Manager Owns this requirement
  Relational Operator : RelationalOperator  Operator===  OutDataTypeStr=boolean
  Scope1 : Scope  NumInputPorts=5
      settings: YMin=-5~-5~-5~-5~-5  YMax=5~5~5~5~5  SaveName=ScopeData5
  Terminator : Terminator
  Terminator1 : Terminator
  wires:
  NtcStInfo/1 -> Scope1/4, Enabled Subsystem/1(In1), Terminator1/1
  NtcNr/1 -> Terminator/1
  NtcSts/1 -> Data Type Conversion1/1
  DebStep/1 -> ISO Fault Debounce Design/2(DebStep), Scope1/2
  ISO Fault Debounce Design/1(Qualifier) -> Relational Operator/1, Scope1/3, Data Store Write/1
  Ground/1 -> ISO Fault Debounce Design/3(SvcClr)
  Data Type Conversion1/1 -> ISO Fault Debounce Design/1(NtcSts), Scope1/1
  ISO Fault Debounce Design/2(ErrAccOut) -> Scope1/5
  Faild/1 -> Relational Operator/2
  Relational Operator/1 -> Enabled Subsystem/Enable

== system CM340A_AdcDiagc/AdcDiagc/AdcDiagcPer1/NTC Fault Processing1/Atomic Subsystem ==
  NtcStInfo : Inport  OutDataTypeStr=uint8
  CopyRight2 : Subsystem  Description=|  mask(Copyright Information){none=on}
      | Copyright info block.                                               
      |                                                                     
      | Place copyright information at the top of every subsystem in design.
      mask prompts: none "No parameters"
      mask help: Place copyright information at the top of every subsystem in design.
      mask Display:
      | NxtrConf = 'Nexteer Confidential';
      | 
      | sys = bdroot; %handle for the current model ("system")
      | first = get_param(sys,'Created');
      | first = first(end-3:end);  %year is last four digits
      | 
      | last = get_param(sys,'LastModifiedDate');
      | if isempty(last)
      |     last = datestr(now,'yyyy');
      | else
      |     last = last(end-3:end);
      | end
      | 
      | if strcmp(first,last)
      |     fprintf('%s -- Copyright %s Nexteer',NxtrConf,first)
      | else
      |     fprintf('%s -- %s%s- %s Nexteer',NxtrConf,char(169),first,last)
      | end
  Fail Step : Subsystem  TreatAsAtomicUnit=on
  If : If
  Merge : Merge
  Merge1 : Merge
  Pass Step : Subsystem  RequirementInfo={} %GIDa_8179ac39_d4c7_4151_9d94_184fec5ce1ce  TreatAsAtomicUnit=on
  NtcSts : Outport
  DebStep : Outport  Port=2  OutDataTypeStr=uint16
  wires:
  Pass Step/2(DebStep) -> Merge/2
  Fail Step/2(DebStep) -> Merge/1
  Merge1/1 -> NtcSts/1
  Pass Step/1(NtcSts) -> Merge1/2
  Fail Step/1(NtcSts) -> Merge1/1
  Merge/1 -> DebStep/1
  If/2 -> Pass Step/Action
  If/1 -> Fail Step/Action
  NtcStInfo/1 -> If/1

== system CM340A_AdcDiagc/AdcDiagc/AdcDiagcPer1/NTC Fault Processing1/CopyRight2 ==

== system CM340A_AdcDiagc/AdcDiagc/AdcDiagcPer1/NTC Fault Processing1/GetNtcQlfr ==
  NtcNr : Inport
  CopyRight2 : Subsystem  Description=|  mask(Copyright Information){none=on}
      | Copyright info block.                                               
      |                                                                     
      | Place copyright information at the top of every subsystem in design.
      mask prompts: none "No parameters"
      mask help: Place copyright information at the top of every subsystem in design.
      mask Display:
      | NxtrConf = 'Nexteer Confidential';
      | 
      | sys = bdroot; %handle for the current model ("system")
      | first = get_param(sys,'Created');
      | first = first(end-3:end);  %year is last four digits
      | 
      | last = get_param(sys,'LastModifiedDate');
      | if isempty(last)
      |     last = datestr(now,'yyyy');
      | else
      |     last = last(end-3:end);
      | end
      | 
      | if strcmp(first,last)
      |     fprintf('%s -- Copyright %s Nexteer',NxtrConf,first)
      | else
      |     fprintf('%s -- %s%s- %s Nexteer',NxtrConf,char(169),first,last)
      | end
  Data Store Read : DataStoreRead  DataStoreName=Adc1DynDiagcQlfr
  Terminator : Terminator
  NtcQlfr : Outport
  wires:
  Data Store Read/1 -> NtcQlfr/1
  NtcNr/1 -> Terminator/1

== system CM340A_AdcDiagc/AdcDiagc/AdcDiagcPer1/NTC Fault Processing1/SetNtcSts ==
  note: Note:
      |
      | - "ISO Fault Debounce Design" Simulink block intent to use here for Simulation purpose only. Do not Code this block
  NtcNr : Inport
  NtcStInfo : Inport  Port=2
  NtcSts : Inport  Port=3  OutDataTypeStr=Enum: NtcSts1
  DebStep : Inport  Port=4
  CopyRight2 : Subsystem  Description=|  mask(Copyright Information){none=on}
      | Copyright info block.                                               
      |                                                                     
      | Place copyright information at the top of every subsystem in design.
      mask prompts: none "No parameters"
      mask help: Place copyright information at the top of every subsystem in design.
      mask Display:
      | NxtrConf = 'Nexteer Confidential';
      | 
      | sys = bdroot; %handle for the current model ("system")
      | first = get_param(sys,'Created');
      | first = first(end-3:end);  %year is last four digits
      | 
      | last = get_param(sys,'LastModifiedDate');
      | if isempty(last)
      |     last = datestr(now,'yyyy');
      | else
      |     last = last(end-3:end);
      | end
      | 
      | if strcmp(first,last)
      |     fprintf('%s -- Copyright %s Nexteer',NxtrConf,first)
      | else
      |     fprintf('%s -- %s%s- %s Nexteer',NxtrConf,char(169),first,last)
      | end
  Data Store Write : DataStoreWrite  DataStoreName=Adc1DynDiagcQlfr
  Data Type Conversion1 : DataTypeConversion  OutMin=0  OutMax=255  OutDataTypeStr=uint8
  Enabled Subsystem : Subsystem  TreatAsAtomicUnit=on
  Faild : Constant  Value=2
  Ground : Ground
  ISO Fault Debounce Design : Stateflow chart  TreatAsAtomicUnit=on
      settings: AttributesFormatString=|
      | Simulation Purpose Only.
      | Do Not Code this block
      | Diagnostic Manager Owns this requirement
  Relational Operator : RelationalOperator  Operator===  OutDataTypeStr=boolean
  Scope1 : Scope  NumInputPorts=5
      settings: YMin=-5~-5~-5~-5~-5  YMax=5~5~5~5~5  SaveName=ScopeData5
  Terminator : Terminator
  Terminator1 : Terminator
  wires:
  ISO Fault Debounce Design/2(ErrAccOut) -> Scope1/5
  Data Type Conversion1/1 -> Scope1/1, ISO Fault Debounce Design/1(NtcSts)
  Ground/1 -> ISO Fault Debounce Design/3(SvcClr)
  DebStep/1 -> Scope1/2, ISO Fault Debounce Design/2(DebStep)
  NtcSts/1 -> Data Type Conversion1/1
  NtcNr/1 -> Terminator/1
  NtcStInfo/1 -> Terminator1/1, Enabled Subsystem/1(In1), Scope1/4
  ISO Fault Debounce Design/1(Qualifier) -> Data Store Write/1, Scope1/3, Relational Operator/1
  Faild/1 -> Relational Operator/2
  Relational Operator/1 -> Enabled Subsystem/Enable

== system CM340A_AdcDiagc/AdcDiagc/AdcDiagcPer1/Adc Daigc Pointer/Strt & End Ptr Output/CopyRight2 ==

== system CM340A_AdcDiagc/AdcDiagc/AdcDiagcPer1/Adc Daigc Pointer/Strt & End Ptr Store/CopyRight2 ==

== system CM340A_AdcDiagc/AdcDiagc/AdcDiagcPer1/Adc Daigc Pointer/Strt & End Ptr Store/State 0 ==
  Action Port : ActionPort  ActionType=then
  Constant3 : Constant  Value=VIRTCH22_CNT_U08
  Constant4 : Constant  Value=VIRTCH23_CNT_U08
  CopyRight2 : Subsystem  Description=|  mask(Copyright Information){none=on}
      | Copyright info block.                                               
      |                                                                     
      | Place copyright information at the top of every subsystem in design.
      mask prompts: none "No parameters"
      mask help: Place copyright information at the top of every subsystem in design.
      mask Display:
      | NxtrConf = 'Nexteer Confidential';
      | 
      | sys = bdroot; %handle for the current model ("system")
      | first = get_param(sys,'Created');
      | first = first(end-3:end);  %year is last four digits
      | 
      | last = get_param(sys,'LastModifiedDate');
      | if isempty(last)
      |     last = datestr(now,'yyyy');
      | else
      |     last = last(end-3:end);
      | end
      | 
      | if strcmp(first,last)
      |     fprintf('%s -- Copyright %s Nexteer',NxtrConf,first)
      | else
      |     fprintf('%s -- %s%s- %s Nexteer',NxtrConf,char(169),first,last)
      | end
  AdcDiagcStrtPtr : Outport
  AdcDiagcEndPtr : Outport  Port=2
  wires:
  Constant3/1 -> AdcDiagcStrtPtr/1
  Constant4/1 -> AdcDiagcEndPtr/1

== system CM340A_AdcDiagc/AdcDiagc/AdcDiagcPer1/Adc Daigc Pointer/Strt & End Ptr Store/State 1 ==
  note: /*Do Nothing*/
  Action Port : ActionPort  ActionType=else
  CopyRight2 : Subsystem  Description=|  mask(Copyright Information){none=on}
      | Copyright info block.                                               
      |                                                                     
      | Place copyright information at the top of every subsystem in design.
      mask prompts: none "No parameters"
      mask help: Place copyright information at the top of every subsystem in design.
      mask Display:
      | NxtrConf = 'Nexteer Confidential';
      | 
      | sys = bdroot; %handle for the current model ("system")
      | first = get_param(sys,'Created');
      | first = first(end-3:end);  %year is last four digits
      | 
      | last = get_param(sys,'LastModifiedDate');
      | if isempty(last)
      |     last = datestr(now,'yyyy');
      | else
      |     last = last(end-3:end);
      | end
      | 
      | if strcmp(first,last)
      |     fprintf('%s -- Copyright %s Nexteer',NxtrConf,first)
      | else
      |     fprintf('%s -- %s%s- %s Nexteer',NxtrConf,char(169),first,last)
      | end

== system CM340A_AdcDiagc/AdcDiagc/AdcDiagcPer1/Adc Daigc Pointer/Strt & End Ptr Store/State 2 ==
  Action Port : ActionPort  ActionType=elseif
  Constant3 : Constant  Value=VIRTCH23_CNT_U08
  Constant4 : Constant  Value=VIRTCH23_CNT_U08
  CopyRight2 : Subsystem  Description=|  mask(Copyright Information){none=on}
      | Copyright info block.                                               
      |                                                                     
      | Place copyright information at the top of every subsystem in design.
      mask prompts: none "No parameters"
      mask help: Place copyright information at the top of every subsystem in design.
      mask Display:
      | NxtrConf = 'Nexteer Confidential';
      | 
      | sys = bdroot; %handle for the current model ("system")
      | first = get_param(sys,'Created');
      | first = first(end-3:end);  %year is last four digits
      | 
      | last = get_param(sys,'LastModifiedDate');
      | if isempty(last)
      |     last = datestr(now,'yyyy');
      | else
      |     last = last(end-3:end);
      | end
      | 
      | if strcmp(first,last)
      |     fprintf('%s -- Copyright %s Nexteer',NxtrConf,first)
      | else
      |     fprintf('%s -- %s%s- %s Nexteer',NxtrConf,char(169),first,last)
      | end
  AdcDiagcStrtPtr : Outport
  AdcDiagcEndPtr : Outport  Port=2
  wires:
  Constant3/1 -> AdcDiagcStrtPtr/1
  Constant4/1 -> AdcDiagcEndPtr/1
